simulink model "BCM_Team"  (R2020b)
settings: Solver=VariableStepAuto  StartTime=0.0  StopTime=10.0  RelTol=1e-3
undefined symbols (not defined in the file or in its folder): sigbuilder_block
libraries: simulink x15, dspswit3 x1
settings Model: Creator=Training  LastModifiedBy=Training

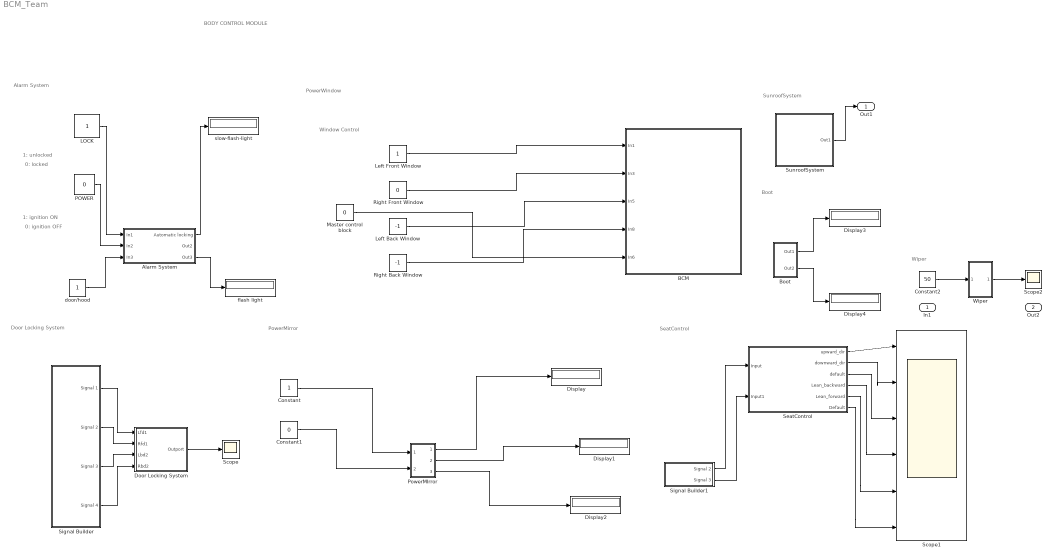
== system BCM_Team ==
  note: BODY CONTROL MODULE
  note: Wiper
  note: Boot
  note: SunroofSystem
  note: SeatControl
  note: PowerMirror
  note: PowerWindow
  note: Door Locking System
  note: Alarm System
  note: 0: locked
  note: 1: unlocked
  note: 1: ignition ON
  note: 0: ignition OFF
  note: Window Control
  In1 : Inport
  " Alarm System" : Subsystem
  BCM : Subsystem
  Boot : Subsystem
  Constant : Constant
  Constant1 : Constant  Value=0
  Constant2 : Constant  Value=50
  Display{,1..4} (5 alike) : Display
  Door Locking System : Subsystem
  LOCK : Constant
      mask Display: image('C:\Users\Training\Desktop\thU1GGBG80.jpg');
  Left Back Window : Constant  Value=-1
  Left Front Window : Constant
  Master control block : Constant  Value=0
  POWER : Constant  Value=0
      mask Display: image('C:\Users\Training\Desktop\power.jpg');
  PowerMIrror : Subsystem
  Right Back Window : Constant  Value=-1
  Right Front Window : Constant  Value=0
  Scope : Scope
  Scope1 : Scope  NumInputPorts=6
  Scope2 : Scope
  SeatControl : Subsystem
  Signal Builder : Subsystem  Tag=STV Subsys  LoadFcn=sigbuilder_block('load');  StartFcn=sigbuilder_block('start');  StopFcn=sigbuilder_block('stop');  ClipboardFcn=sigbuilder_block('clipboard');  mask(Sigbuilder block){tuvar=[0:10]}
      mask help: Simulink:masks:SigbuilderBlock_MD
      mask init:
      | if ~strcmp(get_param(bdroot(gcbh),'SimulationStatus'),'stopped') tuvar = sigbuilder_block('maskInit'); end
      settings: CopyFcn=sigbuilder_block('copy');  DeleteFcn=sigbuilder_block('delete');  ModelCloseFcn=sigbuilder_block('modelClose');  PreSaveFcn=sigbuilder_block('preSave');  PauseFcn=sigbuilder_block('pause');  ContinueFcn=sigbuilder_block('continue');  NameChangeFcn=sigbuilder_block('namechange');  OpenFcn=sigbuilder_block('open',[437.6 199.2 550.4 400 ]);  CloseFcn=sigbuilder_block('close');
      mask Display: plot(0, 0, 100, 100,[2, 2, 32, 32, 2], [68, 8, 8, 68, 68],[32, 2], [38, 38], [32, 19, 2],[53, 60, 44], [32, 17, 17, 2],[16, 16, 31, 31]);txt = getActiveGroup(gcbh);text(2, 100, txt,'verticalAlignment', 'top');
  Signal Builder1 : Subsystem  Tag=STV Subsys  LoadFcn=sigbuilder_block('load');  StartFcn=sigbuilder_block('start');  StopFcn=sigbuilder_block('stop');  ClipboardFcn=sigbuilder_block('clipboard');  mask(Sigbuilder block){tuvar=[0:10]}
      mask help: Simulink:masks:SigbuilderBlock_MD
      mask init:
      | if ~strcmp(get_param(bdroot(gcbh),'SimulationStatus'),'stopped') tuvar = sigbuilder_block('maskInit'); end
      settings: CopyFcn=sigbuilder_block('copy');  DeleteFcn=sigbuilder_block('delete');  ModelCloseFcn=sigbuilder_block('modelClose');  PreSaveFcn=sigbuilder_block('preSave');  PauseFcn=sigbuilder_block('pause');  ContinueFcn=sigbuilder_block('continue');  NameChangeFcn=sigbuilder_block('namechange');  OpenFcn=sigbuilder_block('open',[153.75 66.75 550.5 399.75 ]);  CloseFcn=sigbuilder_block('close');
      mask Display: plot(0, 0, 100, 100,[2, 2, 32, 32, 2], [68, 8, 8, 68, 68],[32, 2], [38, 38], [32, 19, 2],[53, 60, 44], [32, 17, 17, 2],[16, 16, 31, 31]);txt = getActiveGroup(gcbh);text(2, 100, txt,'verticalAlignment', 'top');
  SunroofSystem : Subsystem
      mask Display: image('C:\Users\Training\Downloads\maxresdefault.jpg'); % Use "Edit Image" on toolstrip to change.
  Wiper : Subsystem
  "door/hood " : Constant
  flash light : Display
  slow-flash-light : Display
  Out1 : Outport
  Out2 : Outport  Port=2
  wires:
  LOCK/1 -> " Alarm System"/1(In1)
  POWER/1 -> " Alarm System"/2(In2)
  "door/hood "/1 -> " Alarm System"/3(In3)
  " Alarm System"/1(Automatic locking) -> slow-flash-light/1
  " Alarm System"/3(Out3) -> flash light/1
  Signal Builder/1(Signal 1) -> Door Locking System/1(Lfd1)
  Signal Builder/2(Signal 2) -> Door Locking System/2(Rfd1)
  Signal Builder/3(Signal 3) -> Door Locking System/3(Lbd2)
  Signal Builder/4(Signal 4) -> Door Locking System/4(Rbd2)
  Door Locking System/1(Outport) -> Scope/1
  Right Back Window/1 -> BCM/4(In8)
  Left Back Window/1 -> BCM/3(In5)
  Right Front Window/1 -> BCM/2(In3)
  Left Front Window/1 -> BCM/1(In1)
  Master control block/1 -> BCM/5(In6)
  Constant/1 -> PowerMIrror/1(In1)
  Constant1/1 -> PowerMIrror/2(In2)
  PowerMIrror/1(Out1) -> Display/1
  PowerMIrror/2(Out2) -> Display1/1
  PowerMIrror/3(Out3) -> Display2/1
  SeatControl/5(Lean_forward) -> Scope1/5
  SeatControl/1(upward_dir) -> Scope1/1
  SeatControl/4(Lean_backward) -> Scope1/4
  Signal Builder1/1(Signal 2) -> SeatControl/1(Input)
  Signal Builder1/2(Signal 3) -> SeatControl/2(Input1)
  SeatControl/6(Default) -> Scope1/6
  SeatControl/3(default) -> Scope1/3
  SeatControl/2(downward_dir) -> Scope1/2
  SunroofSystem/1(Out1) -> Out1/1
  Boot/1(Out1) -> Display3/1
  Boot/2(Out2) -> Display4/1
  Wiper/1(Out1) -> Scope2/1
  Constant2/1 -> Wiper/1(In1)

== system BCM_Team/ Alarm System ==
  In1 : Inport
  In2 : Inport  Port=2
  In3 : Inport  Port=3
  Automatic locking system : Subsystem
  Subsystem : Subsystem
  Automatic locking : Outport
  Out2 : Outport  Port=2
  Out3 : Outport  Port=3
  wires:
  Automatic locking system/1(Automatic locking) -> Automatic locking/1, Subsystem/1(In1)
  In3/1 -> Subsystem/2(In2)
  Automatic locking system/2(Out2) -> Out2/1
  Subsystem/1(Out1) -> Out3/1
  In1/1 -> Automatic locking system/1(In1)
  In2/1 -> Automatic locking system/2(In2)

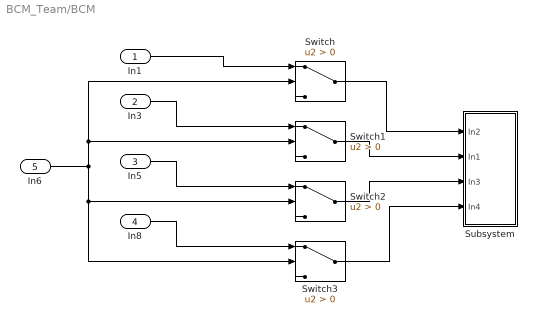
== system BCM_Team/BCM ==
  In1 : Inport
  In3 : Inport  Port=2
  In5 : Inport  Port=3
  In8 : Inport  Port=4
  In6 : Inport  Port=5
  Subsystem : Subsystem
  Switch{,1..3} (4 alike) : Switch  Criteria=u2 > Threshold
  wires:
  In8/1 -> Switch3/1
  In6/1 -> Switch/2, Switch1/2, Switch3/2, Switch2/2
  Switch/1 -> Subsystem/1(In2)
  In3/1 -> Switch1/1
  Switch1/1 -> Subsystem/2(In1)
  In5/1 -> Switch2/1
  Switch3/1 -> Subsystem/4(In4)
  Switch2/1 -> Subsystem/3(In3)
  In1/1 -> Switch/1

== system BCM_Team/Boot ==
  Boot Button Subsystem : Subsystem
  Foot Sensor Subsystem : Subsystem
  Obstacle Detection : Constant
  Out1 : Outport
  Out2 : Outport  Port=2
  wires:
  Obstacle Detection/1 -> Foot Sensor Subsystem/1(In1), Boot Button Subsystem/1(In1)
  Foot Sensor Subsystem/1(Out1) -> Out1/1
  Boot Button Subsystem/1(Out1) -> Out2/1

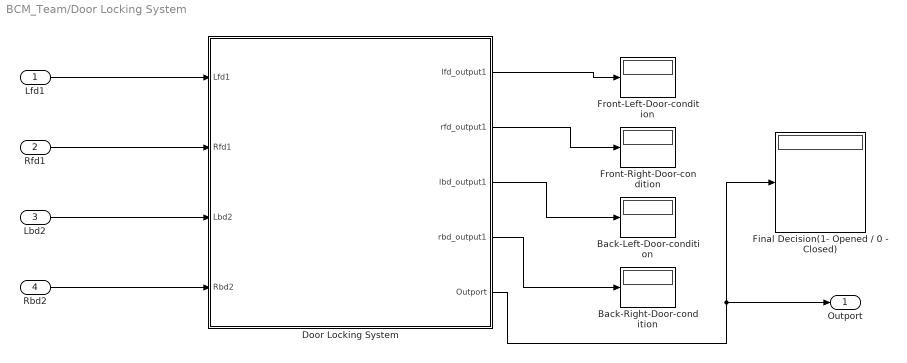
== system BCM_Team/Door Locking System ==
  Lfd1 : Inport
  Rfd1 : Inport  Port=2
  Lbd2 : Inport  Port=3
  Rbd2 : Inport  Port=4
  Back-Left-Door-condition : Display
  Back-Right-Door-condition : Display
  Door Locking System : Subsystem
      mask Display: image('C:\Users\Training\Desktop\asfsf.jpg'); % Use "Edit Image" on toolstrip to change.
  Final Decision(1- Opened / 0 - Closed) : Display
  Front-Left-Door-condition : Display
  Front-Right-Door-condition : Display
  Outport : Outport
  wires:
  Door Locking System/2(rfd_output1) -> Front-Right-Door-condition/1
  Door Locking System/3(lbd_output1) -> Back-Left-Door-condition/1
  Rbd2/1 -> Door Locking System/4(Rbd2)
  Door Locking System/5(Outport) -> Outport/1, Final Decision(1- Opened / 0 - Closed)/1
  Lfd1/1 -> Door Locking System/1(Lfd1)
  Rfd1/1 -> Door Locking System/2(Rfd1)
  Door Locking System/1(lfd_output1) -> Front-Left-Door-condition/1
  Door Locking System/4(rbd_output1) -> Back-Right-Door-condition/1
  Lbd2/1 -> Door Locking System/3(Lbd2)

== system BCM_Team/PowerMIrror ==
  In1 : Inport
  In2 : Inport  Port=2
  OR : Logic  Operator=OR  IconShape=distinctive  AllPortsSameDT=off  OutDataTypeStr=boolean
  Subsystem : Subsystem
      settings: PortSchema="{\"entries\":[{\"content\":{\"sides\":[{\"content\":{\"connectorIds\":[]},\"type\":\"ConnectorPlacement.EquallySpacedRectSide\",\"uuid\":\"24dbb584-65d0-4dd9-8920-8205f0b13d01\"},{\"content\":{\"connectorIds\":[\"Out1\"],\"side\":\"RIGHT\"},\"type\":\"ConnectorPlacement.EquallySpacedRectSide\",\"uuid\":\"108aa5af-9177-456b-a443-ec2af7dc3265\"},{\"content\":{\"connectorIds\":[\"In1\"],\"side\":\"TOP\"},\"type\":\"ConnectorPlacement.EquallySpacedRectSide\",\"uuid\":\"5c407c8d-45ff-4b3c-b030-ff803cb5da46\"},{\"content\":{\"connectorIds\":[],\"side\":\"HIDDEN\"},\"type\":\"ConnectorPlacement.EquallySpacedRectSide\",\"uuid\":\"ff58af5e-ac44-4e34-9293-fa9070ab7545\"}]},\"type\":\"ConnectorPlacement.EquallySpacedConnector\",\"uuid\":\"fb2c6366-9d05-4222-a30c-aebdf7436130\"}],\"packageUris\":[\"http://schema.mathworks.com/mf0/Connector/R2020b\"],\"version\":\"1.0\"}"
  Subsystem1 : Subsystem
  Out1 : Outport
  Out2 : Outport  Port=2
  Out3 : Outport  Port=3
  wires:
  In2/1 -> OR/2
  OR/1 -> Subsystem1/1(In1), Out1/1, Subsystem/1(In1)
  Subsystem/1(Out1) -> Out2/1
  In1/1 -> OR/1
  Subsystem1/1(Out1) -> Out3/1

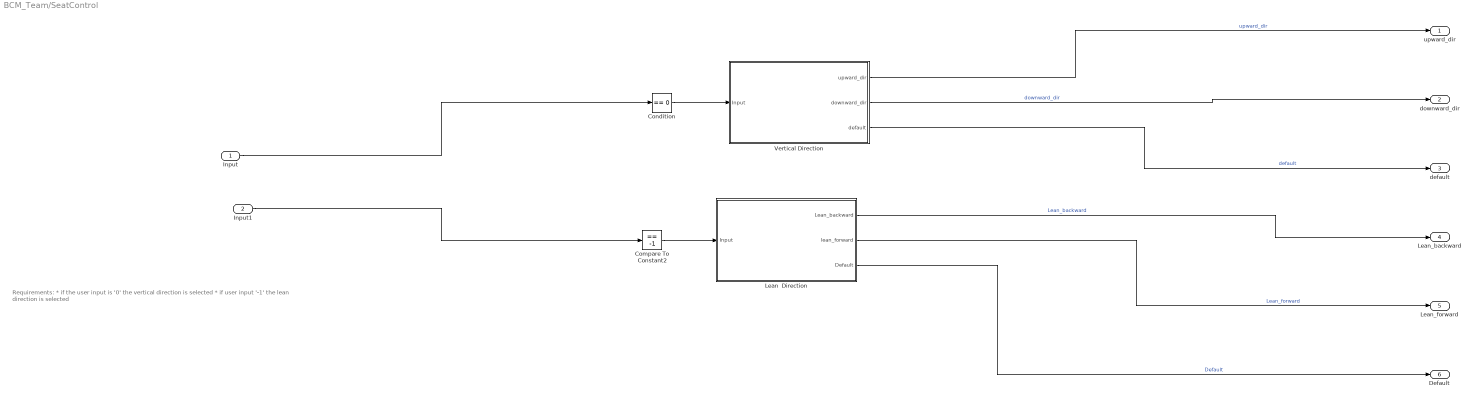
== system BCM_Team/SeatControl ==
  note: Requirements:
      |
      | * if the user input is '0' the vertical direction is selected
      |
      | * if user input '-1' the lean direction is selected
  Input : Inport
  Input1 : Inport  Port=2
  Compare To Constant2 : simulink/Logic and Bit Operations/Compare To Constant  relop===  const=-1  OutDataTypeStr=uint8
  Condition : simulink/Logic and Bit Operations/Compare To Constant  relop===  const=0  OutDataTypeStr=uint8
  Lean  Direction : Subsystem
  Vertical Direction : Subsystem
  upward_dir : Outport
  downward_dir : Outport  Port=2
  default : Outport  Port=3
  Lean_backward : Outport  Port=4
  Lean_forward : Outport  Port=5
  Default : Outport  Port=6
  wires:
  Lean  Direction/3(Default) -> Default/1  "Default"
  Lean  Direction/1(Lean_backward) -> Lean_backward/1  "Lean_backward"
  Condition/1 -> Vertical Direction/1(Input)
  Lean  Direction/2(lean_forward) -> Lean_forward/1  "Lean_forward"
  Compare To Constant2/1 -> Lean  Direction/1(Input)
  Vertical Direction/3(default) -> default/1  "default"
  Input1/1 -> Compare To Constant2/1
  Vertical Direction/1(upward_dir) -> upward_dir/1  "upward_dir"
  Input/1 -> Condition/1
  Vertical Direction/2(downward_dir) -> downward_dir/1  "downward_dir"

== system BCM_Team/Signal Builder ==
  Demux : Demux  Tag=STV Demux
      settings: DisplayOption=none
  FromWs : FromWorkspace  Tag=STV FromWs  VariableName=tuvar
      SigBuilderData=|
      | common.afterFinalStr = 'Extrapolate'
      | common.sampleTime = 0
      | dataSet.timeRange = [0 10]
      | dataSet.name = 'Group 1'
      | sbobj.Groups.Name = 'Group 1'
      | sbobj.Groups.Signals(1).Name = 'Signal 1'
      | sbobj.Groups.Signals(1).XData = [0 4 4 6 6 10]
      | sbobj.Groups.Signals(1).YData = [0 0 1 1 0 0]
      | sbobj.Groups.Signals(2).Name = 'Signal 2'
      | sbobj.Groups.Signals(2).XData = [0 5 5 10]
      | sbobj.Groups.Signals(2).YData = [0 0 1 1]
      | sbobj.Groups.Signals(3).Name = 'Signal 3'
      | sbobj.Groups.Signals(3).XData = [0 4 4 6 6 10]
      | sbobj.Groups.Signals(3).YData = [0 0 1 1 0 0]
      | sbobj.Groups.Signals(4).Name = 'Signal 4'
      | sbobj.Groups.Signals(4).XData = [0 5 5 10]
      | sbobj.Groups.Signals(4).YData = [0 0 1 1]
  Signal 1 : Outport  Tag=STV Outport
  Signal 2 : Outport  Tag=STV Outport  Port=2
  Signal 3 : Outport  Tag=STV Outport  Port=3
  Signal 4 : Outport  Tag=STV Outport  Port=4
  wires:
  Demux/1 -> Signal 1/1
  FromWs/1 -> Demux/1
  Demux/2 -> Signal 2/1
  Demux/3 -> Signal 3/1
  Demux/4 -> Signal 4/1

== system BCM_Team/Signal Builder1 ==
  Demux : Demux  Tag=STV Demux  Outputs=2
      settings: DisplayOption=none
  FromWs : FromWorkspace  Tag=STV FromWs  VariableName=tuvar
      SigBuilderData=|
      | common.afterFinalStr = 'Extrapolate'
      | common.sampleTime = 0
      | dataSet.timeRange = [0 10]
      | dataSet.name = 'Group 1'
      | sbobj.Groups.Name = 'Group 1'
      | sbobj.Groups.Signals(1).Name = 'Signal 2'
      | sbobj.Groups.Signals(1).XData = [0 10]
      | sbobj.Groups.Signals(1).YData = [0 0]
      | sbobj.Groups.Signals(2).Name = 'Signal 3'
      | sbobj.Groups.Signals(2).XData = [0 10]
      | sbobj.Groups.Signals(2).YData = [-1 -1]
  Signal 2 : Outport  Tag=STV Outport
  Signal 3 : Outport  Tag=STV Outport  Port=2
  wires:
  FromWs/1 -> Demux/1
  Demux/1 -> Signal 2/1
  Demux/2 -> Signal 3/1

== system BCM_Team/SunroofSystem ==
  Constant : Constant  Value=30
  Constant2 : Constant  Value=31.7483455882353
  Slider : SliderBlock  ScaleMax=40
  Switch : Switch  Criteria=u2 > Threshold  Threshold=30
  Out1 : Outport
  wires:
  Constant/1 -> Switch/1
  Constant2/1 -> Switch/2, Switch/3
  Switch/1 -> Out1/1

== system BCM_Team/Wiper ==
  note: low
  In1 : Inport
  Merge : Merge  Inputs=4
  Signal Builder : Subsystem  Tag=STV Subsys  LoadFcn=sigbuilder_block('load');  StartFcn=sigbuilder_block('start');  StopFcn=sigbuilder_block('stop');  ClipboardFcn=sigbuilder_block('clipboard');  mask(Sigbuilder block){tuvar=[0:10]}
      mask help: Simulink:masks:SigbuilderBlock_MD
      mask init:
      | if ~strcmp(get_param(bdroot(gcbh),'SimulationStatus'),'stopped') tuvar = sigbuilder_block('maskInit'); end
      settings: CopyFcn=sigbuilder_block('copy');  DeleteFcn=sigbuilder_block('delete');  ModelCloseFcn=sigbuilder_block('modelClose');  PreSaveFcn=sigbuilder_block('preSave');  PauseFcn=sigbuilder_block('pause');  ContinueFcn=sigbuilder_block('continue');  NameChangeFcn=sigbuilder_block('namechange');  OpenFcn=sigbuilder_block('open',[437.6 199.2 550.4 400 ]);  CloseFcn=sigbuilder_block('close');
      mask Display: plot(0, 0, 100, 100,[2, 2, 32, 32, 2], [68, 8, 8, 68, 68],[32, 2], [38, 38], [32, 19, 2],[53, 60, 44], [32, 17, 17, 2],[16, 16, 31, 31]);txt = getActiveGroup(gcbh);text(2, 100, txt,'verticalAlignment', 'top');
  Switch Case Action Subsystem : Subsystem  TreatAsAtomicUnit=on
  Switch Case Action Subsystem1 : Subsystem  TreatAsAtomicUnit=on
  Switch Case Action Subsystem2 : Subsystem  TreatAsAtomicUnit=on
  Switch Case Action Subsystem3 : Subsystem  TreatAsAtomicUnit=on
  threshold_comparison : If  IfExpression=u1<=10  ElseIfExpressions=u1<=30,u1<=50
  Out1 : Outport
  wires:
  Switch Case Action Subsystem2/1(Out1) -> Merge/3
  threshold_comparison/4 -> Switch Case Action Subsystem3/Action  "high"
  threshold_comparison/3 -> Switch Case Action Subsystem2/Action  "medium"
  Signal Builder/1(Signal 1) -> Switch Case Action Subsystem/1(In1)
  Signal Builder/4(Signal 4) -> Switch Case Action Subsystem3/1(In1)
  Switch Case Action Subsystem1/1(Out1) -> Merge/2
  Signal Builder/3(Signal 3) -> Switch Case Action Subsystem2/1(In1)
  threshold_comparison/1 -> Switch Case Action Subsystem/Action  "off"
  In1/1 -> threshold_comparison/1
  threshold_comparison/2 -> Switch Case Action Subsystem1/Action
  Switch Case Action Subsystem/1(Out1) -> Merge/1
  Switch Case Action Subsystem3/1(Out1) -> Merge/4
  Signal Builder/2(Signal 2) -> Switch Case Action Subsystem1/1(In1)
  Merge/1 -> Out1/1

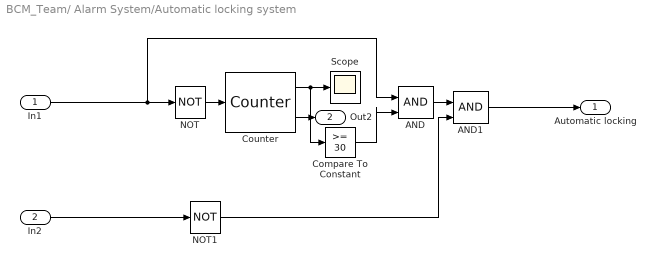
== system BCM_Team/ Alarm System/Automatic locking system ==
  In1 : Inport
  In2 : Inport  Port=2
  AND : Logic  IconShape=distinctive  AllPortsSameDT=off  OutDataTypeStr=boolean
  AND1 : Logic  IconShape=distinctive  AllPortsSameDT=off  OutDataTypeStr=boolean
  Compare To Constant : simulink/Logic and Bit Operations/Compare To Constant  relop=>=  const=30  OutDataTypeStr=boolean
  Counter : dspswit3/Counter  Direction=Up  CountEvent=Free running  CounterSize=32 bits  MaxCount=300  InitialCount=30  Output=Count and Hit  HitValue=32  ResetInput=on  SamplesPerFrame=1  Ts=1  CntDtype=double  HitDtype=Logical
  NOT : Logic  Operator=NOT  IconShape=distinctive  AllPortsSameDT=off  OutDataTypeStr=boolean
  NOT1 : Logic  Operator=NOT  IconShape=distinctive  AllPortsSameDT=off  OutDataTypeStr=boolean
  Scope : Scope
  Automatic locking : Outport
  Out2 : Outport  Port=2
  wires:
  NOT/1 -> Counter/1
  Counter/1 -> Compare To Constant/1, Scope/1
  In2/1 -> NOT1/1
  AND/1 -> AND1/1
  AND1/1 -> Automatic locking/1
  Counter/2 -> Out2/1
  In1/1 -> AND/1, NOT/1
  Compare To Constant/1 -> AND/2
  NOT1/1 -> AND1/2

== system BCM_Team/ Alarm System/Subsystem ==
  In1 : Inport
  In2 : Inport  Port=2
  AND : Logic  IconShape=distinctive  AllPortsSameDT=off  OutDataTypeStr=boolean
  Constant1 : Constant
  NOT : Logic  Operator=NOT  IconShape=distinctive  AllPortsSameDT=off  OutDataTypeStr=boolean
  Switch : Switch  Criteria=u2 > Threshold
  Out1 : Outport
  wires:
  AND/1 -> Switch/2
  NOT/1 -> Switch/3
  Constant1/1 -> NOT/1, Switch/1
  In1/1 -> AND/1
  In2/1 -> AND/2
  Switch/1 -> Out1/1

== system BCM_Team/BCM/Subsystem ==
  In2 : Inport
  In1 : Inport  Port=2
  In3 : Inport  Port=3
  In4 : Inport  Port=4
  Left_B : Subsystem
  Left_F : Subsystem
  Right_B : Subsystem
  Right_F : Subsystem
  wires:
  In4/1 -> ?
  In1/1 -> Left_B/1(In1)
  In2/1 -> Right_F/1(In1)
  In3/1 -> ?

== system BCM_Team/Boot/Boot Button Subsystem ==
  In1 : Inport
  Boot Button : Constant
  Constant3 : Constant
  Constant4 : Constant
  OR : Logic  IconShape=distinctive  AllPortsSameDT=off  OutDataTypeStr=boolean
  Switch : Switch
  Out1 : Outport
  wires:
  Constant4/1 -> OR/1
  Constant3/1 -> Switch/1
  Switch/1 -> Out1/1
  Boot Button/1 -> OR/2
  OR/1 -> Switch/2
  In1/1 -> Switch/3

== system BCM_Team/Boot/Foot Sensor Subsystem ==
  In1 : Inport
  Constant : Constant
  Constant1 : Constant
  Foot Sensor : Constant
  OR1 : Logic  IconShape=distinctive  AllPortsSameDT=off  OutDataTypeStr=boolean
  Switch1 : Switch  ZeroCross=off
  Out1 : Outport
  wires:
  Constant1/1 -> Switch1/1
  Foot Sensor/1 -> OR1/2
  In1/1 -> Switch1/3
  OR1/1 -> Switch1/2
  Constant/1 -> OR1/1
  Switch1/1 -> Out1/1

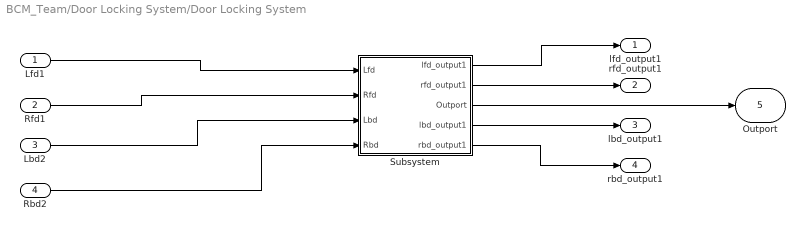
== system BCM_Team/Door Locking System/Door Locking System ==
  Lfd1 : Inport
  Rfd1 : Inport  Port=2
  Lbd2 : Inport  Port=3
  Rbd2 : Inport  Port=4
  Subsystem : Subsystem
  lfd_output1 : Outport
  rfd_output1 : Outport  Port=2
  lbd_output1 : Outport  Port=3
  rbd_output1 : Outport  Port=4
  Outport : Outport  Port=5
  wires:
  Subsystem/2(rfd_output1) -> rfd_output1/1
  Lfd1/1 -> Subsystem/1(Lfd)
  Subsystem/1(lfd_output1) -> lfd_output1/1
  Subsystem/5(rbd_output1) -> rbd_output1/1
  Subsystem/4(lbd_output1) -> lbd_output1/1
  Rfd1/1 -> Subsystem/2(Rfd)
  Lbd2/1 -> Subsystem/3(Lbd)
  Rbd2/1 -> Subsystem/4(Rbd)
  Subsystem/3(Outport) -> Outport/1

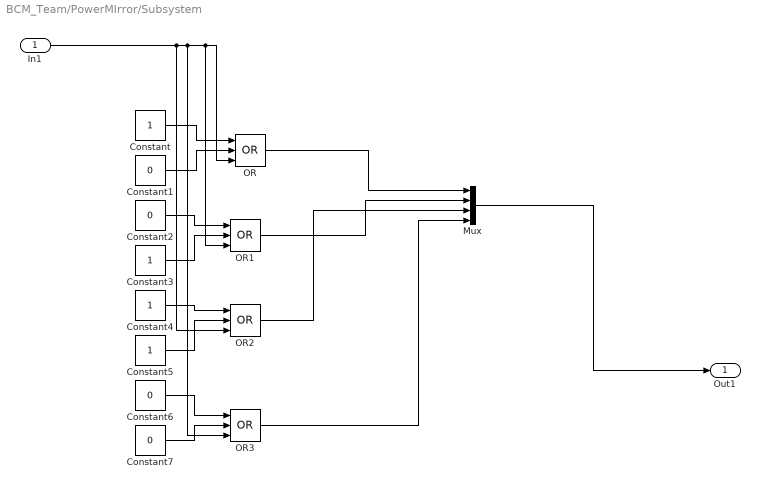
== system BCM_Team/PowerMIrror/Subsystem ==
  In1 : Inport
  Constant{,3..5} (4 alike) : Constant
  Constant{1..2,6..7} (4 alike) : Constant  Value=0
  Mux : Mux
  OR{,1..3} (4 alike) : Logic  Operator=OR  Inputs=3  IconShape=distinctive  AllPortsSameDT=off  OutDataTypeStr=boolean
  Out1 : Outport
  wires:
  Constant/1 -> OR/1
  Constant1/1 -> OR/2
  Constant2/1 -> OR1/1
  Constant3/1 -> OR1/2
  Constant4/1 -> OR2/1
  Constant5/1 -> OR2/2
  Constant6/1 -> OR3/1
  Constant7/1 -> OR3/2
  OR/1 -> Mux/1
  OR1/1 -> Mux/2
  OR2/1 -> Mux/3
  OR3/1 -> Mux/4
  Mux/1 -> Out1/1
  In1/1 -> OR2/3, OR3/3, OR1/3, OR/3

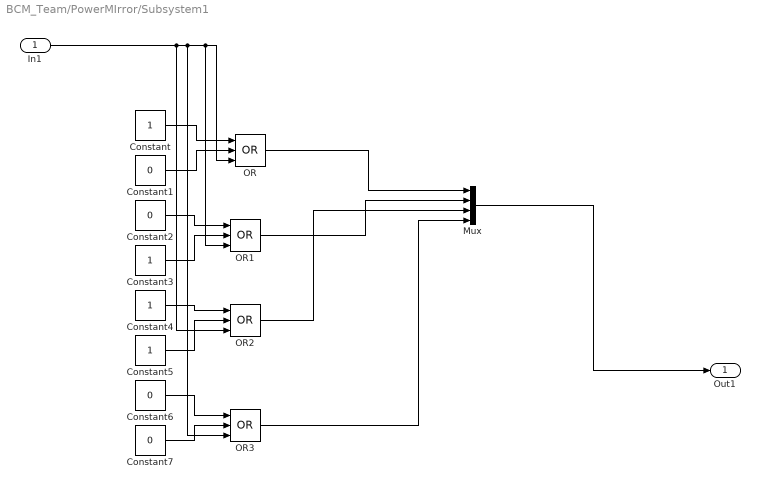
== system BCM_Team/PowerMIrror/Subsystem1 ==
  In1 : Inport
  Constant{,3..5} (4 alike) : Constant
  Constant{1..2,6..7} (4 alike) : Constant  Value=0
  Mux : Mux
  OR{,1..3} (4 alike) : Logic  Operator=OR  Inputs=3  IconShape=distinctive  AllPortsSameDT=off  OutDataTypeStr=boolean
  Out1 : Outport
  wires:
  Constant/1 -> OR/1
  Constant1/1 -> OR/2
  Constant2/1 -> OR1/1
  Constant3/1 -> OR1/2
  Constant4/1 -> OR2/1
  Constant5/1 -> OR2/2
  Constant6/1 -> OR3/1
  Constant7/1 -> OR3/2
  OR/1 -> Mux/1
  OR1/1 -> Mux/2
  OR2/1 -> Mux/3
  OR3/1 -> Mux/4
  Mux/1 -> Out1/1
  In1/1 -> OR2/3, OR3/3, OR1/3, OR/3

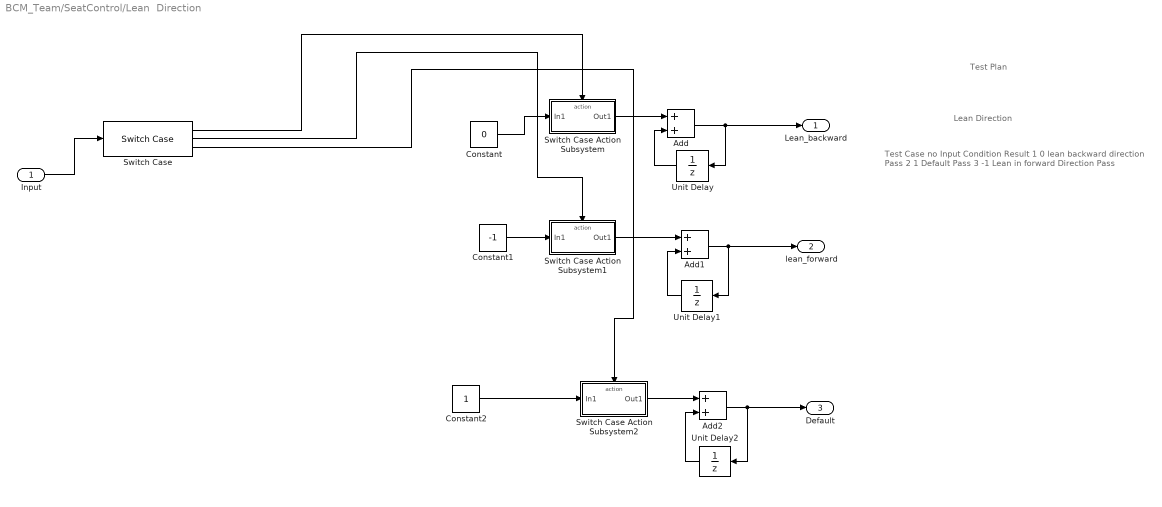
== system BCM_Team/SeatControl/Lean  Direction ==
  note: Lean Direction
  note: Test Plan
  note: Test Case no
      | Input
      | Condition
      | Result
      |
      | 1
      | 0
      | lean backward direction
      | Pass
      |
      | 2
      | 1
      | Default
      | Pass
      |
      | 3
      | -1
      | Lean in forward Direction
      | Pass
  Input : Inport
  Add : Sum
  Add1 : Sum
  Add2 : Sum
  Constant : Constant  Value=0
  Constant1 : Constant  Value=-1
  Constant2 : Constant
  Switch Case : SwitchCase  CaseConditions={0,-1}
  Switch Case Action Subsystem : Subsystem  TreatAsAtomicUnit=on
  Switch Case Action Subsystem1 : Subsystem  TreatAsAtomicUnit=on
  Switch Case Action Subsystem2 : Subsystem  TreatAsAtomicUnit=on
  Unit Delay : UnitDelay  SampleTime=-1  HasFrameUpgradeWarning=on
  Unit Delay1 : UnitDelay  SampleTime=-1  HasFrameUpgradeWarning=on
  Unit Delay2 : UnitDelay  SampleTime=-1  HasFrameUpgradeWarning=on
  Lean_backward : Outport
  lean_forward : Outport  Port=2
  Default : Outport  Port=3
  wires:
  Add1/1 -> lean_forward/1, Unit Delay1/1
  Constant1/1 -> Switch Case Action Subsystem1/1(In1)
  Input/1 -> Switch Case/1
  Constant2/1 -> Switch Case Action Subsystem2/1(In1)
  Unit Delay2/1 -> Add2/2
  Switch Case Action Subsystem1/1(Out1) -> Add1/1
  Add2/1 -> Default/1, Unit Delay2/1
  Unit Delay1/1 -> Add1/2
  Switch Case/1 -> Switch Case Action Subsystem/Action
  Add/1 -> Lean_backward/1, Unit Delay/1
  Switch Case Action Subsystem/1(Out1) -> Add/1
  Constant/1 -> Switch Case Action Subsystem/1(In1)
  Unit Delay/1 -> Add/2
  Switch Case/3 -> Switch Case Action Subsystem2/Action
  Switch Case Action Subsystem2/1(Out1) -> Add2/1
  Switch Case/2 -> Switch Case Action Subsystem1/Action

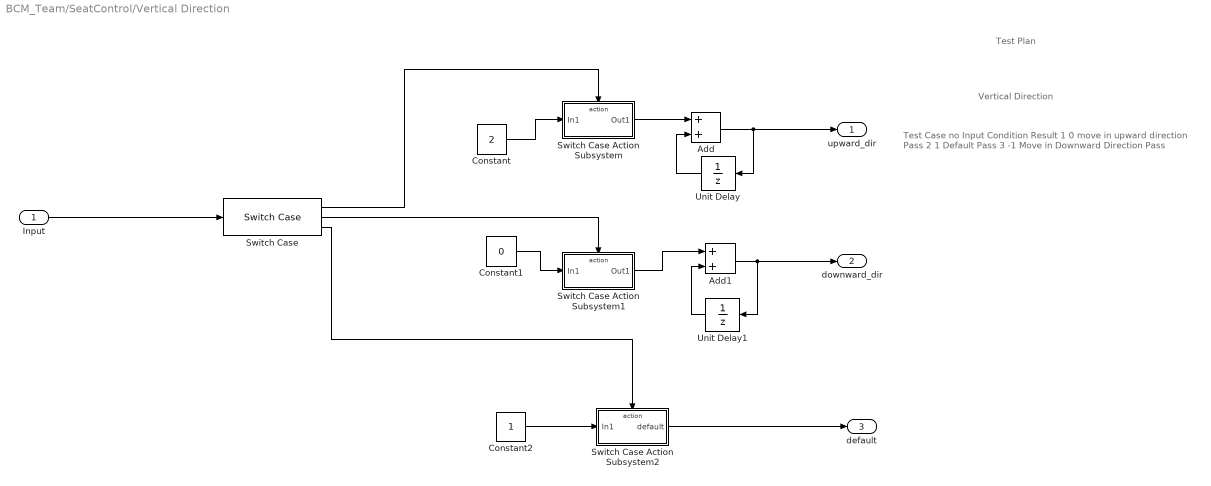
== system BCM_Team/SeatControl/Vertical Direction ==
  note: Test Plan
  note: Vertical Direction
  note: Test Case no
      | Input
      | Condition
      | Result
      |
      | 1
      | 0
      | move in upward direction
      | Pass
      |
      | 2
      | 1
      | Default
      | Pass
      |
      | 3
      | -1
      | Move in Downward Direction
      | Pass
  Input : Inport
  Add : Sum
  Add1 : Sum
  Constant : Constant  Value=2
  Constant1 : Constant  Value=0
  Constant2 : Constant
  Switch Case : SwitchCase  CaseConditions={0,-1}
  Switch Case Action Subsystem : Subsystem  TreatAsAtomicUnit=on
  Switch Case Action Subsystem1 : Subsystem  TreatAsAtomicUnit=on
  Switch Case Action Subsystem2 : Subsystem  TreatAsAtomicUnit=on
  Unit Delay : UnitDelay  SampleTime=-1  HasFrameUpgradeWarning=on
  Unit Delay1 : UnitDelay  SampleTime=-1  HasFrameUpgradeWarning=on
  upward_dir : Outport
  downward_dir : Outport  Port=2
  default : Outport  Port=3
  wires:
  Add1/1 -> downward_dir/1, Unit Delay1/1
  Constant1/1 -> Switch Case Action Subsystem1/1(In1)
  Input/1 -> Switch Case/1
  Constant2/1 -> Switch Case Action Subsystem2/1(In1)
  Switch Case Action Subsystem1/1(Out1) -> Add1/1
  Switch Case Action Subsystem2/1(default) -> default/1
  Unit Delay1/1 -> Add1/2
  Switch Case/1 -> Switch Case Action Subsystem/Action
  Add/1 -> upward_dir/1, Unit Delay/1
  Switch Case Action Subsystem/1(Out1) -> Add/1
  Constant/1 -> Switch Case Action Subsystem/1(In1)
  Unit Delay/1 -> Add/2
  Switch Case/3 -> Switch Case Action Subsystem2/Action
  Switch Case/2 -> Switch Case Action Subsystem1/Action

== system BCM_Team/Wiper/Signal Builder ==
  Demux : Demux  Tag=STV Demux
      settings: DisplayOption=none
  FromWs : FromWorkspace  Tag=STV FromWs  VariableName=tuvar
      SigBuilderData=|
      | common.afterFinalStr = 'Extrapolate'
      | common.sampleTime = 0
      | dataSet.timeRange = [0 10]
      | dataSet.name = 'Group 1'
      | sbobj.Groups.Name = 'Group 1'
      | sbobj.Groups.Signals(1).Name = 'Signal 1'
      | sbobj.Groups.Signals(1).XData = [0 4 4 6 6 10]
      | sbobj.Groups.Signals(1).YData = [0 0 1 1 0 0]
      | sbobj.Groups.Signals(2).Name = 'Signal 2'
      | sbobj.Groups.Signals(2).XData = [0 0.5 0.5 1 1 1.5 1.5 2 2 2.5 2.5 3 3 3.5 3.5 4 4 4.5 4.5 5 5 5.5 5.5 6 6 6.5 6.5 7 7 7.5 7.5 8 8 8.5 8.5 9 9 9.5 9.5 10]
      | sbobj.Groups.Signals(2).YData = [2 2 0 0 2 2 0 0 2 2 0 0 2 2 0 0 2 2 0 0 2 2 0 0 2 2 0 0 2 2 0 0 2 2 0 0 2 2 0 0]
      | sbobj.Groups.Signals(3).Name = 'Signal 3'
      | sbobj.Groups.Signals(3).XData = [0 1 1 2 2 3 3 4 4 5 5 6 6 7 7 8 8 9 9 10]
      | sbobj.Groups.Signals(3).YData = [0 2 0 2 0 2 0 2 0 2 0 2 0 2 0 2 0 2 0 2]
      | sbobj.Groups.Signals(4).Name = 'Signal 4'
      | sbobj.Groups.Signals(4).XData = [0 5 5 10]
      | sbobj.Groups.Signals(4).YData = [0 0 1 1]
  Signal 1 : Outport  Tag=STV Outport
  Signal 2 : Outport  Tag=STV Outport  Port=2
  Signal 3 : Outport  Tag=STV Outport  Port=3
  Signal 4 : Outport  Tag=STV Outport  Port=4
  wires:
  Demux/1 -> Signal 1/1
  FromWs/1 -> Demux/1
  Demux/2 -> Signal 2/1
  Demux/3 -> Signal 3/1
  Demux/4 -> Signal 4/1

== system BCM_Team/Wiper/Switch Case Action Subsystem ==
  In1 : Inport
  Action Port : ActionPort
  Out1 : Outport
  wires:
  In1/1 -> Out1/1

== system BCM_Team/Wiper/Switch Case Action Subsystem1 ==
  In1 : Inport
  Action Port : ActionPort
  Out1 : Outport
  wires:
  In1/1 -> Out1/1

== system BCM_Team/Wiper/Switch Case Action Subsystem2 ==
  In1 : Inport
  Action Port : ActionPort
  Out1 : Outport
  wires:
  In1/1 -> Out1/1

== system BCM_Team/Wiper/Switch Case Action Subsystem3 ==
  In1 : Inport
  Action Port : ActionPort
  Out1 : Outport
  wires:
  In1/1 -> Out1/1

== system BCM_Team/BCM/Subsystem/Left_B ==
  In1 : Inport
  Add : Sum
  Button not pressed : Constant  Value=0
  Constant1 : Constant
  Motor_LF : Scope  NumInputPorts=2
  RampSignal1 : simulink/Sources/Ramp  slope=1  start=0  InitialOutput=0
  RampSignal2 : simulink/Sources/Ramp  slope=1  start=0  InitialOutput=0
  Start : Subsystem  Tag=STV Subsys  LoadFcn=sigbuilder_block('load');  StartFcn=sigbuilder_block('start');  StopFcn=sigbuilder_block('stop');  ClipboardFcn=sigbuilder_block('clipboard');  mask(Sigbuilder block){tuvar=[0:10]}
      mask help: Simulink:masks:SigbuilderBlock_MD
      mask init:
      | if ~strcmp(get_param(bdroot(gcbh),'SimulationStatus'),'stopped') tuvar = sigbuilder_block('maskInit'); end
      settings: CopyFcn=sigbuilder_block('copy');  DeleteFcn=sigbuilder_block('delete');  ModelCloseFcn=sigbuilder_block('modelClose');  PreSaveFcn=sigbuilder_block('preSave');  PauseFcn=sigbuilder_block('pause');  ContinueFcn=sigbuilder_block('continue');  NameChangeFcn=sigbuilder_block('namechange');  OpenFcn=sigbuilder_block('open',[437.6 199.2 550.4 400 ]);  CloseFcn=sigbuilder_block('close');
      mask Display: plot(0, 0, 100, 100,[2, 2, 32, 32, 2], [68, 8, 8, 68, 68],[32, 2], [38, 38], [32, 19, 2],[53, 60, 44], [32, 17, 17, 2],[16, 16, 31, 31]);txt = getActiveGroup(gcbh);text(2, 100, txt,'verticalAlignment', 'top');
  Window DOWN_LF : Switch
  Window UP_LF : Switch  Criteria=u2 > Threshold
  wires:
  Add/1 -> Window DOWN_LF/2
  Button not pressed/1 -> Window UP_LF/3, Window DOWN_LF/3
  Constant1/1 -> Add/2
  RampSignal2/1 -> Window DOWN_LF/1
  Window DOWN_LF/1 -> Motor_LF/2
  Start/1(Signal 1) -> Add/1, Window UP_LF/2
  RampSignal1/1 -> Window UP_LF/1
  Window UP_LF/1 -> Motor_LF/1

== system BCM_Team/BCM/Subsystem/Left_F ==
  Add : Sum
  Button not pressed : Constant  Value=0
  Constant1 : Constant
  Motor_LF : Scope  NumInputPorts=2
  RampSignal1 : simulink/Sources/Ramp  slope=1  start=0  InitialOutput=0
  RampSignal2 : simulink/Sources/Ramp  slope=1  start=0  InitialOutput=0
  Start : Subsystem  Tag=STV Subsys  LoadFcn=sigbuilder_block('load');  StartFcn=sigbuilder_block('start');  StopFcn=sigbuilder_block('stop');  ClipboardFcn=sigbuilder_block('clipboard');  mask(Sigbuilder block){tuvar=[0:10]}
      mask help: Simulink:masks:SigbuilderBlock_MD
      mask init:
      | if ~strcmp(get_param(bdroot(gcbh),'SimulationStatus'),'stopped') tuvar = sigbuilder_block('maskInit'); end
      settings: CopyFcn=sigbuilder_block('copy');  DeleteFcn=sigbuilder_block('delete');  ModelCloseFcn=sigbuilder_block('modelClose');  PreSaveFcn=sigbuilder_block('preSave');  PauseFcn=sigbuilder_block('pause');  ContinueFcn=sigbuilder_block('continue');  NameChangeFcn=sigbuilder_block('namechange');  OpenFcn=sigbuilder_block('open',[437.6 199.2 550.4 400 ]);  CloseFcn=sigbuilder_block('close');
      mask Display: plot(0, 0, 100, 100,[2, 2, 32, 32, 2], [68, 8, 8, 68, 68],[32, 2], [38, 38], [32, 19, 2],[53, 60, 44], [32, 17, 17, 2],[16, 16, 31, 31]);txt = getActiveGroup(gcbh);text(2, 100, txt,'verticalAlignment', 'top');
  Window DOWN_LF : Switch
  "Window UP_LF " : Switch  Criteria=u2 > Threshold
  wires:
  Add/1 -> Window DOWN_LF/2
  Button not pressed/1 -> "Window UP_LF "/3, Window DOWN_LF/3
  Constant1/1 -> Add/2
  RampSignal2/1 -> Window DOWN_LF/1
  Window DOWN_LF/1 -> Motor_LF/2
  Start/1(Signal 1) -> Add/1, "Window UP_LF "/2
  RampSignal1/1 -> "Window UP_LF "/1
  "Window UP_LF "/1 -> Motor_LF/1

== system BCM_Team/BCM/Subsystem/Right_B ==
  Add : Sum
  Button not pressed : Constant  Value=0
  Constant1 : Constant
  Motor_RB : Scope  NumInputPorts=2
  Ramp signal : simulink/Sources/Ramp  slope=1  start=0  InitialOutput=0
  Ramp signal 1 : simulink/Sources/Ramp  slope=1  start=0  InitialOutput=0
  Start : Subsystem  Tag=STV Subsys  LoadFcn=sigbuilder_block('load');  StartFcn=sigbuilder_block('start');  StopFcn=sigbuilder_block('stop');  ClipboardFcn=sigbuilder_block('clipboard');  mask(Sigbuilder block){tuvar=[0:10]}
      mask help: Simulink:masks:SigbuilderBlock_MD
      mask init:
      | if ~strcmp(get_param(bdroot(gcbh),'SimulationStatus'),'stopped') tuvar = sigbuilder_block('maskInit'); end
      settings: CopyFcn=sigbuilder_block('copy');  DeleteFcn=sigbuilder_block('delete');  ModelCloseFcn=sigbuilder_block('modelClose');  PreSaveFcn=sigbuilder_block('preSave');  PauseFcn=sigbuilder_block('pause');  ContinueFcn=sigbuilder_block('continue');  NameChangeFcn=sigbuilder_block('namechange');  OpenFcn=sigbuilder_block('open',[437.6 199.2 550.4 400 ]);  CloseFcn=sigbuilder_block('close');
      mask Display: plot(0, 0, 100, 100,[2, 2, 32, 32, 2], [68, 8, 8, 68, 68],[32, 2], [38, 38], [32, 19, 2],[53, 60, 44], [32, 17, 17, 2],[16, 16, 31, 31]);txt = getActiveGroup(gcbh);text(2, 100, txt,'verticalAlignment', 'top');
  Window DOWN_RB : Switch
  Window UP_RB : Switch  Criteria=u2 > Threshold
  wires:
  Add/1 -> Window DOWN_RB/2
  Button not pressed/1 -> Window UP_RB/3, Window DOWN_RB/3
  Constant1/1 -> Add/2
  Ramp signal/1 -> Window DOWN_RB/1
  Window DOWN_RB/1 -> Motor_RB/2
  Start/1(Signal 1) -> Add/1, Window UP_RB/2
  Ramp signal 1/1 -> Window UP_RB/1
  Window UP_RB/1 -> Motor_RB/1

== system BCM_Team/BCM/Subsystem/Right_F ==
  In1 : Inport
  Add : Sum
  Button not pressed : Constant  Value=0
  Constant1 : Constant
  Motor_RF : Scope  NumInputPorts=2
  RampSignal1 : simulink/Sources/Ramp  slope=1  start=0  InitialOutput=0
  RampSignal2 : simulink/Sources/Ramp  slope=1  start=0  InitialOutput=0
  Start : Subsystem  Tag=STV Subsys  LoadFcn=sigbuilder_block('load');  StartFcn=sigbuilder_block('start');  StopFcn=sigbuilder_block('stop');  ClipboardFcn=sigbuilder_block('clipboard');  mask(Sigbuilder block){tuvar=[0:10]}
      mask help: Simulink:masks:SigbuilderBlock_MD
      mask init:
      | if ~strcmp(get_param(bdroot(gcbh),'SimulationStatus'),'stopped') tuvar = sigbuilder_block('maskInit'); end
      settings: CopyFcn=sigbuilder_block('copy');  DeleteFcn=sigbuilder_block('delete');  ModelCloseFcn=sigbuilder_block('modelClose');  PreSaveFcn=sigbuilder_block('preSave');  PauseFcn=sigbuilder_block('pause');  ContinueFcn=sigbuilder_block('continue');  NameChangeFcn=sigbuilder_block('namechange');  OpenFcn=sigbuilder_block('open',[437.6 199.2 550.4 400 ]);  CloseFcn=sigbuilder_block('close');
      mask Display: plot(0, 0, 100, 100,[2, 2, 32, 32, 2], [68, 8, 8, 68, 68],[32, 2], [38, 38], [32, 19, 2],[53, 60, 44], [32, 17, 17, 2],[16, 16, 31, 31]);txt = getActiveGroup(gcbh);text(2, 100, txt,'verticalAlignment', 'top');
  Window DOWN_RF : Switch
  Window UP_RF : Switch  Criteria=u2 > Threshold
  wires:
  Add/1 -> Window DOWN_RF/2
  Button not pressed/1 -> Window UP_RF/3, Window DOWN_RF/3
  Constant1/1 -> Add/2
  RampSignal2/1 -> Window DOWN_RF/1
  Window DOWN_RF/1 -> Motor_RF/2
  Start/1(Signal 1) -> Add/1, Window UP_RF/2
  RampSignal1/1 -> Window UP_RF/1
  Window UP_RF/1 -> Motor_RF/1

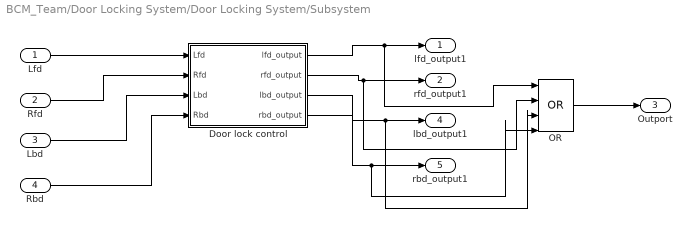
== system BCM_Team/Door Locking System/Door Locking System/Subsystem ==
  Lfd : Inport
  Rfd : Inport  Port=2
  Lbd : Inport  Port=3
  Rbd : Inport  Port=4
  Door lock control : Subsystem
  OR : Logic  Operator=OR  Inputs=4  IconShape=distinctive  AllPortsSameDT=off  OutDataTypeStr=boolean
  lfd_output1 : Outport
  rfd_output1 : Outport  Port=2
  Outport : Outport  Port=3
  lbd_output1 : Outport  Port=4
  rbd_output1 : Outport  Port=5
  wires:
  Door lock control/4(rbd_output) -> rbd_output1/1, OR/4
  Rfd/1 -> Door lock control/2(Rfd)
  Door lock control/2(rfd_output) -> rfd_output1/1, OR/2
  Door lock control/3(lbd_output) -> lbd_output1/1, OR/3
  Lbd/1 -> Door lock control/3(Lbd)
  Door lock control/1(lfd_output) -> lfd_output1/1, OR/1
  Lfd/1 -> Door lock control/1(Lfd)
  Rbd/1 -> Door lock control/4(Rbd)
  OR/1 -> Outport/1

== system BCM_Team/SeatControl/Lean  Direction/Switch Case Action Subsystem ==
  In1 : Inport
  Action Port : ActionPort
  Out1 : Outport
  wires:
  In1/1 -> Out1/1

== system BCM_Team/SeatControl/Lean  Direction/Switch Case Action Subsystem1 ==
  In1 : Inport
  Action Port : ActionPort
  Out1 : Outport
  wires:
  In1/1 -> Out1/1

== system BCM_Team/SeatControl/Lean  Direction/Switch Case Action Subsystem2 ==
  In1 : Inport
  Action Port : ActionPort
  Out1 : Outport
  wires:
  In1/1 -> Out1/1

== system BCM_Team/SeatControl/Vertical Direction/Switch Case Action Subsystem ==
  In1 : Inport
  Action Port : ActionPort
  Out1 : Outport
  wires:
  In1/1 -> Out1/1

== system BCM_Team/SeatControl/Vertical Direction/Switch Case Action Subsystem1 ==
  In1 : Inport
  Action Port : ActionPort
  Out1 : Outport
  wires:
  In1/1 -> Out1/1

== system BCM_Team/SeatControl/Vertical Direction/Switch Case Action Subsystem2 ==
  In1 : Inport
  Action Port : ActionPort
  default : Outport
  wires:
  In1/1 -> default/1

== system BCM_Team/BCM/Subsystem/Left_B/Start ==
  Demux : Demux  Tag=STV Demux  Outputs=1
      settings: DisplayOption=none
  FromWs : FromWorkspace  Tag=STV FromWs  VariableName=tuvar
      SigBuilderData=|
      | common.afterFinalStr = 'Extrapolate'
      | common.sampleTime = 0
      | dataSet.timeRange = [0 10]
      | dataSet.name = 'Group 1'
      | sbobj.Groups.Name = 'Group 1'
      | sbobj.Groups.Signals.Name = 'Signal 1'
      | sbobj.Groups.Signals.XData = [0 4 4 6 6 10]
      | sbobj.Groups.Signals.YData = [0 0 1 1 0 0]
  Signal 1 : Outport  Tag=STV Outport
  wires:
  Demux/1 -> Signal 1/1
  FromWs/1 -> Demux/1

== system BCM_Team/BCM/Subsystem/Left_F/Start ==
  Demux : Demux  Tag=STV Demux  Outputs=1
      settings: DisplayOption=none
  FromWs : FromWorkspace  Tag=STV FromWs  VariableName=tuvar
      SigBuilderData=|
      | common.afterFinalStr = 'Extrapolate'
      | common.sampleTime = 0
      | dataSet.timeRange = [0 10]
      | dataSet.name = 'Group 1'
      | sbobj.Groups.Name = 'Group 1'
      | sbobj.Groups.Signals.Name = 'Signal 1'
      | sbobj.Groups.Signals.XData = [0 4 4 6 6 10]
      | sbobj.Groups.Signals.YData = [0 0 1 1 0 0]
  Signal 1 : Outport  Tag=STV Outport
  wires:
  Demux/1 -> Signal 1/1
  FromWs/1 -> Demux/1

== system BCM_Team/BCM/Subsystem/Right_B/Start ==
  Demux : Demux  Tag=STV Demux  Outputs=1
      settings: DisplayOption=none
  FromWs : FromWorkspace  Tag=STV FromWs  VariableName=tuvar
      SigBuilderData=|
      | common.afterFinalStr = 'Extrapolate'
      | common.sampleTime = 0
      | dataSet.timeRange = [0 10]
      | dataSet.name = 'Group 1'
      | sbobj.Groups.Name = 'Group 1'
      | sbobj.Groups.Signals.Name = 'Signal 1'
      | sbobj.Groups.Signals.XData = [0 4 4 6 6 10]
      | sbobj.Groups.Signals.YData = [0 0 1 1 0 0]
  Signal 1 : Outport  Tag=STV Outport
  wires:
  Demux/1 -> Signal 1/1
  FromWs/1 -> Demux/1

== system BCM_Team/BCM/Subsystem/Right_F/Start ==
  Demux : Demux  Tag=STV Demux  Outputs=1
      settings: DisplayOption=none
  FromWs : FromWorkspace  Tag=STV FromWs  VariableName=tuvar
      SigBuilderData=|
      | common.afterFinalStr = 'Extrapolate'
      | common.sampleTime = 0
      | dataSet.timeRange = [0 10]
      | dataSet.name = 'Group 1'
      | sbobj.Groups.Name = 'Group 1'
      | sbobj.Groups.Signals.Name = 'Signal 1'
      | sbobj.Groups.Signals.XData = [0 4 4 6 6 10]
      | sbobj.Groups.Signals.YData = [0 0 1 1 0 0]
  Signal 1 : Outport  Tag=STV Outport
  wires:
  Demux/1 -> Signal 1/1
  FromWs/1 -> Demux/1

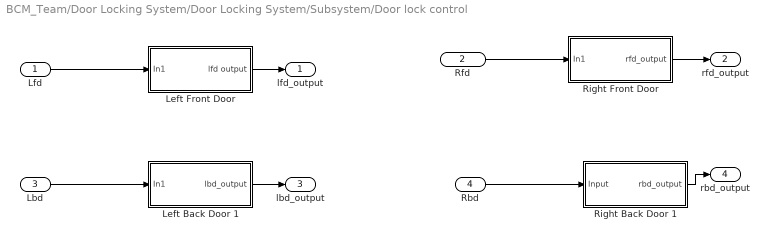
== system BCM_Team/Door Locking System/Door Locking System/Subsystem/Door lock control ==
  Lfd : Inport
  Rfd : Inport  Port=2
  Lbd : Inport  Port=3
  Rbd : Inport  Port=4
  Left Back Door 1 : Subsystem
  "Left Front Door " : Subsystem
  Right Back Door 1 : Subsystem
  "Right Front Door " : Subsystem
  lfd_output : Outport
  rfd_output : Outport  Port=2
  lbd_output : Outport  Port=3
  rbd_output : Outport  Port=4
  wires:
  Lfd/1 -> "Left Front Door "/1(In1)
  "Left Front Door "/1(lfd output) -> lfd_output/1
  Rfd/1 -> "Right Front Door "/1(In1)
  "Right Front Door "/1(rfd_output) -> rfd_output/1
  Lbd/1 -> Left Back Door 1/1(In1)
  Left Back Door 1/1(lbd_output) -> lbd_output/1
  Rbd/1 -> Right Back Door 1/1(Input)
  Right Back Door 1/1(rbd_output) -> rbd_output/1

== system BCM_Team/Door Locking System/Door Locking System/Subsystem/Door lock control/Left Back Door 1 ==
  In1 : Inport
  Constant : Constant  Value=0
  Ramp : simulink/Sources/Ramp  slope=0  start=0  InitialOutput=1
  Switch : Switch  Criteria=u2 > Threshold
  lbd_output : Outport
  wires:
  In1/1 -> Switch/2
  Switch/1 -> lbd_output/1
  Constant/1 -> Switch/3
  Ramp/1 -> Switch/1

== system BCM_Team/Door Locking System/Door Locking System/Subsystem/Door lock control/Left Front Door  ==
  In1 : Inport
  Constant : Constant  Value=0
  Ramp : simulink/Sources/Ramp  slope=0  start=0  InitialOutput=1
  S1 : Switch  Criteria=u2 > Threshold
  lfd output : Outport
  wires:
  In1/1 -> S1/2
  S1/1 -> lfd output/1
  Constant/1 -> S1/3
  Ramp/1 -> S1/1

== system BCM_Team/Door Locking System/Door Locking System/Subsystem/Door lock control/Right Back Door 1 ==
  Input : Inport
  Constant : Constant  Value=0
  Ramp_input : simulink/Sources/Ramp  slope=0  start=0  InitialOutput=1
  Switch : Switch  Criteria=u2 > Threshold
  rbd_output : Outport
  wires:
  Input/1 -> Switch/2
  Switch/1 -> rbd_output/1
  Constant/1 -> Switch/3
  Ramp_input/1 -> Switch/1

== system BCM_Team/Door Locking System/Door Locking System/Subsystem/Door lock control/Right Front Door  ==
  In1 : Inport
  Constant : Constant  Value=0
  Ramp : simulink/Sources/Ramp  slope=0  start=0  InitialOutput=1
  Switch : Switch  Criteria=u2 > Threshold
  rfd_output : Outport
  wires:
  In1/1 -> Switch/2
  Switch/1 -> rfd_output/1
  Constant/1 -> Switch/3
  Ramp/1 -> Switch/1
